simulink model "TP_Robot_Mobile"  (R2024b)
settings: Solver=FixedStepAuto  StartTime=0.0  StopTime=10.0  FixedStep=dt  RelTol=1e-3
undefined symbols (not defined in the file): Km, Kx, Ky, l, L, tau
settings Model: Creator=alessandrini  LastModifiedBy=aalessan

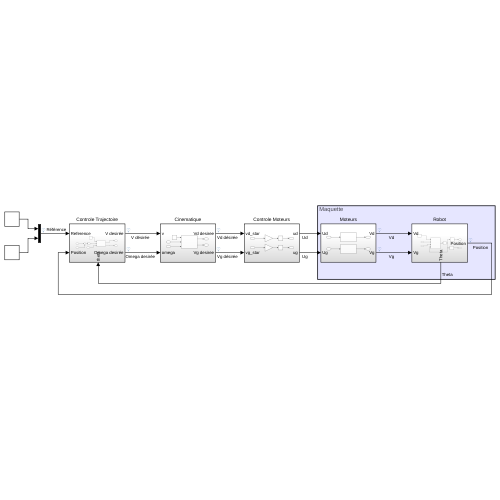
[thumbnail: Simulink's stored preview of the top-level diagram]
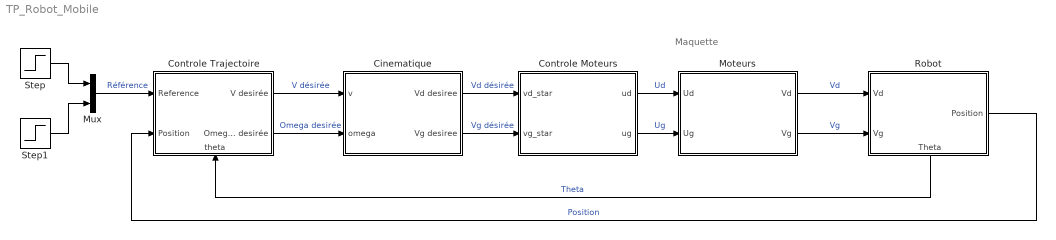
== system TP_Robot_Mobile ==
  note: Maquette
  Cinematique : Subsystem
  Controle Moteurs : Subsystem
  Controle Trajectoire : Subsystem
      settings: PortSchema="{\"entries\":[{\"content\":{\"sides\":[{\"content\":{\"connectorIds\":[\"In1\",\"In2\"]},\"type\":\"ConnectorPlacement.EquallySpacedRectSide\",\"uuid\":\"ef553a2d-daa0-4cfb-8b1d-11cc981dcd73\"},{\"content\":{\"connectorIds\":[\"Out1\",\"Out2\"],\"side\":\"RIGHT\"},\"type\":\"ConnectorPlacement.EquallySpacedRectSide\",\"uuid\":\"4255286a-b82d-4586-8beb-ea79ce4b2519\"},{\"content\":{\"side\":\"TOP\"},\"type\":\"ConnectorPlacement.EquallySpacedRectSide\",\"uuid\":\"5f4898d5-e3e9-457a-8a78-49067b012858\"},{\"content\":{\"connectorIds\":[\"In3\"],\"side\":\"BOTTOM\"},\"type\":\"ConnectorPlacement.EquallySpacedRectSide\",\"uuid\":\"bead9bd8-d65e-4ffb-b0ee-ad8e1e301bef\"}]},\"type\":\"ConnectorPlacement.EquallySpacedConnector\",\"uuid\":\"789b2371-4041-4359-b528-9bc5424f8c42\"}],\"packageUris\":[\"http://schema.mathworks.com/mf0/Connector/R2020b\"],\"version\":\"1.0\"}"
  Moteurs : Subsystem
  Mux : Mux  Inputs=2
  Robot : Subsystem
      settings: PortSchema="{\"entries\":[{\"content\":{\"sides\":[{\"content\":{\"connectorIds\":[\"In1\",\"In2\"]},\"type\":\"ConnectorPlacement.EquallySpacedRectSide\",\"uuid\":\"465d5ee7-5407-4cec-9692-595a507b417d\"},{\"content\":{\"connectorIds\":[\"Out1\"],\"side\":\"RIGHT\"},\"type\":\"ConnectorPlacement.EquallySpacedRectSide\",\"uuid\":\"c2aa6d28-3c59-40b4-8fa5-9570a2fa95d9\"},{\"content\":{\"side\":\"TOP\"},\"type\":\"ConnectorPlacement.EquallySpacedRectSide\",\"uuid\":\"0ba5684a-01dc-44c5-a5cb-386c3cb182f8\"},{\"content\":{\"connectorIds\":[\"Out2\"],\"side\":\"BOTTOM\"},\"type\":\"ConnectorPlacement.EquallySpacedRectSide\",\"uuid\":\"f33bc4cb-898c-4ca7-aa33-083b6855c93e\"}]},\"type\":\"ConnectorPlacement.EquallySpacedConnector\",\"uuid\":\"37bcc828-48b2-4619-96a5-ccb75e3c8e2d\"}],\"packageUris\":[\"http://schema.mathworks.com/mf0/Connector/R2020b\"],\"version\":\"1.0\"}"
  Step : Step  After=150  SampleTime=0
  Step1 : Step  After=150  SampleTime=0
  wires:
  Controle Moteurs/1(ud) -> Moteurs/1(Ud)  "Ud"
  Controle Moteurs/2(ug) -> Moteurs/2(Ug)  "Ug"
  Cinematique/1(Vd desiree) -> Controle Moteurs/1(vd_star)  "Vd désirée"
  Cinematique/2(Vg desiree) -> Controle Moteurs/2(vg_star)  "Vg désirée"
  Controle Trajectoire/1(V desirée) -> Cinematique/1(v)  "V désirée"
  Controle Trajectoire/2(Omega desirée) -> Cinematique/2(omega)  "Omega desirée"
  Robot/1(Position) -> Controle Trajectoire/2(Position)  "Position"
  Moteurs/1(Vd) -> Robot/1(Vd)  "Vd"
  Moteurs/2(Vg) -> Robot/2(Vg)  "Vg"
  Mux/1 -> Controle Trajectoire/1(Reference)  "Référence"
  Step/1 -> Mux/1
  Step1/1 -> Mux/2
  Robot/2(Theta) -> Controle Trajectoire/3(theta)  "Theta"

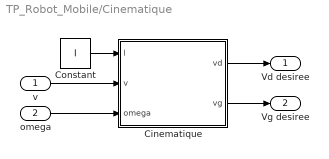
== system TP_Robot_Mobile/Cinematique ==
  v : Inport
  omega : Inport  Port=2
  Cinematique : MATLAB Function  TreatAsAtomicUnit=on
  Constant : Constant  Value=l
  Vd desiree : Outport
  Vg desiree : Outport  Port=2
  wires:
  v/1 -> Cinematique/2(v)
  Cinematique/1(vd) -> Vd desiree/1
  Cinematique/2(vg) -> Vg desiree/1
  omega/1 -> Cinematique/3(omega)
  Constant/1 -> Cinematique/1(l)

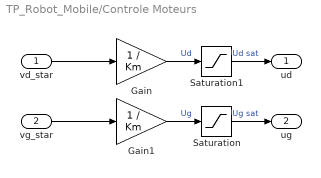
== system TP_Robot_Mobile/Controle Moteurs ==
  vd_star : Inport
  vg_star : Inport  Port=2
  Gain : Gain  Gain=1 / Km
  Gain1 : Gain  Gain=1 / Km
  Saturation : Saturate  UpperLimit=9  LowerLimit=-9
  Saturation1 : Saturate  UpperLimit=9  LowerLimit=-9
  ud : Outport
  ug : Outport  Port=2
  wires:
  Gain/1 -> Saturation1/1  "Ud"
  Gain1/1 -> Saturation/1  "Ug"
  vd_star/1 -> Gain/1
  vg_star/1 -> Gain1/1
  Saturation/1 -> ug/1  "Ug sat"
  Saturation1/1 -> ud/1  "Ud sat"

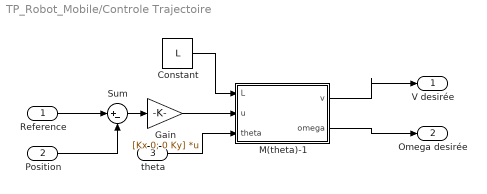
== system TP_Robot_Mobile/Controle Trajectoire ==
  Reference : Inport
  Position : Inport  Port=2
  theta : Inport  Port=3
  Constant : Constant  Value=L
  Gain : Gain  Gain=[Kx 0; 0 Ky]  Multiplication=Matrix(K*u)
  M(theta)-1 : MATLAB Function  TreatAsAtomicUnit=on
  Sum : Sum  Inputs=|+-
  V desirée : Outport
  Omega desirée : Outport  Port=2
  wires:
  M(theta)-1/1(v) -> V desirée/1
  M(theta)-1/2(omega) -> Omega desirée/1
  theta/1 -> M(theta)-1/3(theta)
  Position/1 -> Sum/2
  Reference/1 -> Sum/1
  Sum/1 -> Gain/1
  Gain/1 -> M(theta)-1/2(u)
  Constant/1 -> M(theta)-1/1(L)

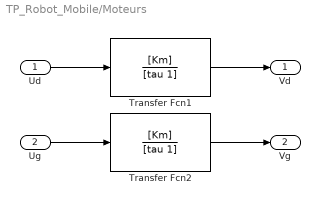
== system TP_Robot_Mobile/Moteurs ==
  Ud : Inport
  Ug : Inport  Port=2
  Transfer Fcn1 : TransferFcn  Numerator=[Km]  Denominator=[tau 1]
  Transfer Fcn2 : TransferFcn  Numerator=[Km]  Denominator=[tau 1]
  Vd : Outport
  Vg : Outport  Port=2
  wires:
  Transfer Fcn1/1 -> Vd/1
  Transfer Fcn2/1 -> Vg/1
  Ug/1 -> Transfer Fcn2/1
  Ud/1 -> Transfer Fcn1/1

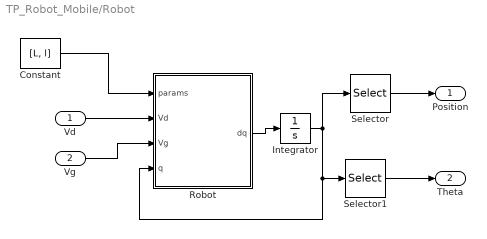
== system TP_Robot_Mobile/Robot ==
  Vd : Inport
  Vg : Inport  Port=2
  Constant : Constant  Value=[L, l]
  Integrator : Integrator
  Robot : MATLAB Function  TreatAsAtomicUnit=on
  Selector : Selector  InputPortWidth=3  IndexOptions=Index vector (dialog)  Indices=[1 2]  OutputSizes=1
  Selector1 : Selector  InputPortWidth=3  IndexOptions=Index vector (dialog)  Indices=[3]  OutputSizes=1
  Position : Outport
  Theta : Outport  Port=2
  wires:
  Selector/1 -> Position/1
  Selector1/1 -> Theta/1
  Integrator/1 -> Robot/4(q), Selector1/1, Selector/1
  Robot/1(dq) -> Integrator/1
  Vd/1 -> Robot/2(Vd)
  Vg/1 -> Robot/3(Vg)
  Constant/1 -> Robot/1(params)

== matlab function TP_Robot_Mobile/Cinematique/Cinematique ==
  data: l input; v input; vd output; omega input; vg output
function [vd, vg]= fcn(l, v, omega)

vd = v + l * omega;
vg = v - l * omega;

== matlab function TP_Robot_Mobile/Robot/Robot ==
  data: params input; Vd input; dq output; Vg input; q input
function dq  = fcn(params, Vd, Vg, q)

L = params(1); l = params(2);
v = (Vd + Vg) / 2; 
omega = (Vd - Vg) / (2 * l);

dq = [cos(q(3)), -L*sin(q(3)); sin(q(3)), L*cos(q(3)); 0, 1] * [v; omega];

== matlab function TP_Robot_Mobile/Controle Trajectoire/M(theta)-1 ==
  data: L input; u input; v output; theta input; omega output
function [v, omega]= fcn(L, u, theta)
    
    ux = u(1); uy = u(2);
    v = ux * cos(theta) + uy * sin(theta);
    omega = 1 / L * (uy * cos(theta) - ux * sin(theta));
